simulink model "BlueROVHeavy_SlidingModeControl"  (R2024b)
settings: Solver=ode45  StartTime=0.0  StopTime=T  FixedStep=Ts  RelTol=1e-3
InitFcn:
  | run BlueRovHeavy_init.m;
values from neighbouring files (symbols this model uses):
  BLUEROV_DATA = struct()    [BlueRovHeavy_data.m]
  Ks_D = 25    [BlueRovHeavy_init.m]
  Ks_S = 4    [BlueRovHeavy_init.m]
  Lambda = 21*eye(6)    [BlueRovHeavy_init.m]
libraries: robotcorelib x1
settings Model: Creator=salva  LastModifiedBy=salva

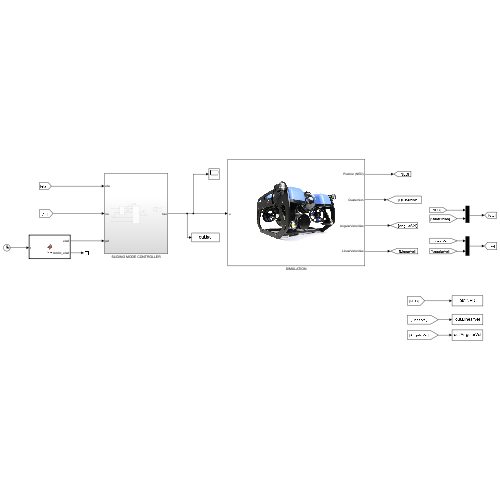
[thumbnail: Simulink's stored preview of the top-level diagram]
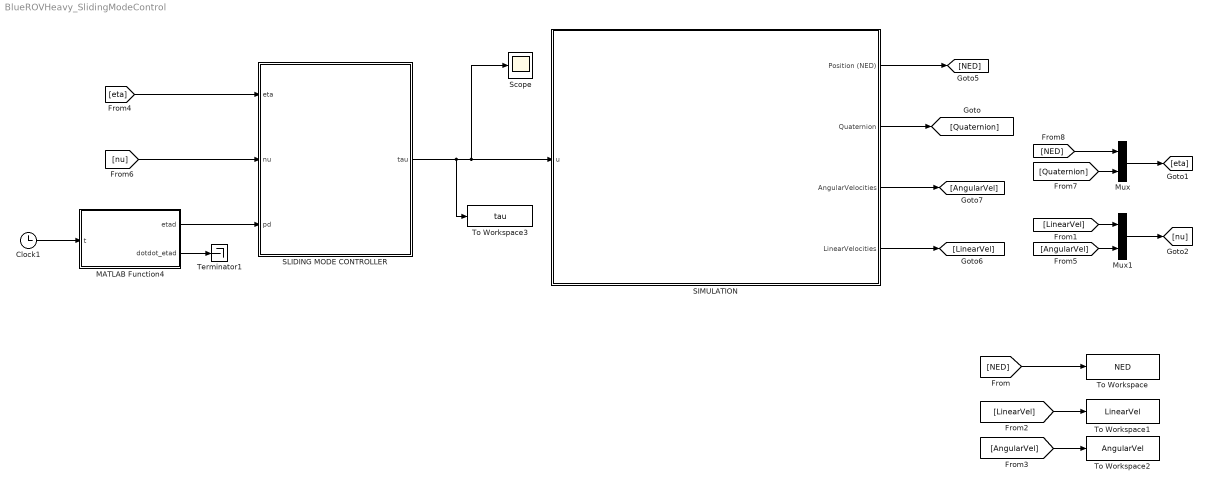
== system BlueROVHeavy_SlidingModeControl ==
  Clock1 : Clock
  MATLAB Function4 : MATLAB Function  TreatAsAtomicUnit=on
  Mux : Mux  Inputs=2
  Mux1 : Mux  Inputs=2
  SIMULATION : Subsystem
      mask Display: image('BlueROVpic.jpg', [0,0,0,0,90,90]);
  SLIDING MODE CONTROLLER : Subsystem
  Scope : Scope
  Terminator1 : Terminator
  To Workspace : ToWorkspace  VariableName=NED  SaveFormat=Timeseries  SampleTime=-1
  To Workspace1 : ToWorkspace  VariableName=LinearVel  SaveFormat=Timeseries  SampleTime=-1
  To Workspace2 : ToWorkspace  VariableName=AngularVel  SaveFormat=Timeseries  SampleTime=-1
  To Workspace3 : ToWorkspace  VariableName=tau  SaveFormat=Timeseries  SampleTime=-1
  wires:
  Mux/1 -> [eta]
  Mux1/1 -> [nu]
  [eta] -> SLIDING MODE CONTROLLER/1(eta)
  [nu] -> SLIDING MODE CONTROLLER/2(nu)
  SLIDING MODE CONTROLLER/1(tau) -> To Workspace3/1, Scope/1, SIMULATION/1(u)
  MATLAB Function4/1(etad) -> SLIDING MODE CONTROLLER/3(pd)
  Clock1/1 -> MATLAB Function4/1(t)
  MATLAB Function4/2(dotdot_etad) -> Terminator1/1
  [NED] -> To Workspace/1
  [AngularVel] -> To Workspace2/1
  [LinearVel] -> To Workspace1/1
  SIMULATION/1(Position (NED)) -> [NED]
  SIMULATION/2(Quaternion) -> [Quaternion]
  [AngularVel] -> Mux1/2
  [LinearVel] -> Mux1/1
  SIMULATION/4(LinearVelocities) -> [LinearVel]
  SIMULATION/3(AngularVelocities) -> [AngularVel]
  [Quaternion] -> Mux/2
  [NED] -> Mux/1

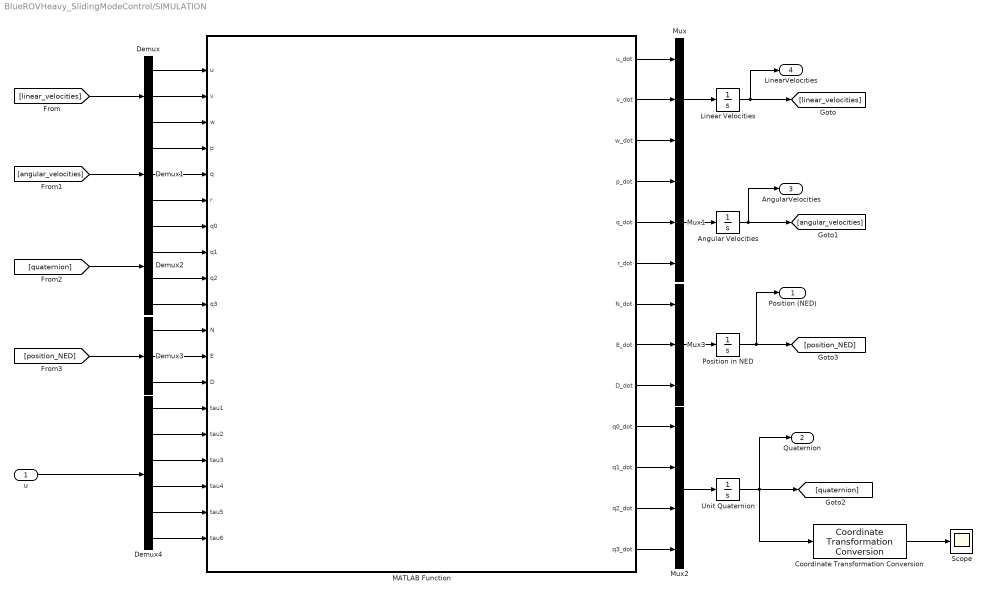
== system BlueROVHeavy_SlidingModeControl/SIMULATION ==
  u : Inport
  Angular Velocities : Integrator  InitialCondition=[0;0;0]  UpperSaturationLimit=50  LowerSaturationLimit=-50
  Coordinate Transformation Conversion : robotcorelib/Coordinate Transformation Conversion  InputRepresentation=Quaternion  InputEulerSequence=ZYX  ShowTrVecInputPort=on  OutputRepresentation=Euler Angles  OutputEulerSequence=XYZ  ShowTrVecOutputPort=on  SimulateUsing=Interpreted execution
  Demux : Demux  Outputs=3
  Demux1 : Demux  Outputs=3
  Demux2 : Demux
  Demux3 : Demux  Outputs=3
  Demux4 : Demux  Outputs=6
  Linear Velocities : Integrator  InitialCondition=[0.1;0;0]
  MATLAB Function : MATLAB Function  TreatAsAtomicUnit=on
  Mux : Mux  Inputs=3
  Mux1 : Mux  Inputs=3
  Mux2 : Mux
  Mux3 : Mux  Inputs=3
  Position in NED : Integrator  InitialCondition=[3;0;9]
  Scope : Scope
  Unit Quaternion : Integrator  InitialCondition=[1,0,0,0]
  Position (NED) : Outport
  Quaternion : Outport  Port=2
  AngularVelocities : Outport  Port=3
  LinearVelocities : Outport  Port=4
  wires:
  Demux1/1 -> MATLAB Function/4(p)
  Demux4/5 -> MATLAB Function/18(tau5)
  Demux1/2 -> MATLAB Function/5(q)
  Demux4/6 -> MATLAB Function/19(tau6)
  Demux/2 -> MATLAB Function/2(v)
  Mux3/1 -> Position in NED/1
  Demux/1 -> MATLAB Function/1(u)
  Demux1/3 -> MATLAB Function/6(r)
  Angular Velocities/1 -> [angular_velocities], AngularVelocities/1
  Demux3/1 -> MATLAB Function/11(N)
  Demux3/3 -> MATLAB Function/13(D)
  Demux4/2 -> MATLAB Function/15(tau2)
  Mux/1 -> Linear Velocities/1
  Mux1/1 -> Angular Velocities/1
  Demux4/4 -> MATLAB Function/17(tau4)
  Demux2/3 -> MATLAB Function/9(q2)
  Demux2/2 -> MATLAB Function/8(q1)
  Demux3/2 -> MATLAB Function/12(E)
  Demux2/1 -> MATLAB Function/7(q0)
  Demux4/1 -> MATLAB Function/14(tau1)
  Demux4/3 -> MATLAB Function/16(tau3)
  Demux/3 -> MATLAB Function/3(w)
  [linear_velocities] -> Demux/1
  [angular_velocities] -> Demux1/1
  [quaternion] -> Demux2/1
  [position_NED] -> Demux3/1
  u/1 -> Demux4/1
  MATLAB Function/1(u_dot) -> Mux/1
  MATLAB Function/2(v_dot) -> Mux/2
  MATLAB Function/3(w_dot) -> Mux/3
  Linear Velocities/1 -> [linear_velocities], LinearVelocities/1
  MATLAB Function/4(p_dot) -> Mux1/1
  MATLAB Function/5(q_dot) -> Mux1/2
  MATLAB Function/6(r_dot) -> Mux1/3
  MATLAB Function/7(N_dot) -> Mux3/1
  MATLAB Function/8(E_dot) -> Mux3/2
  MATLAB Function/9(D_dot) -> Mux3/3
  MATLAB Function/10(q0_dot) -> Mux2/1
  MATLAB Function/11(q1_dot) -> Mux2/2
  MATLAB Function/12(q2_dot) -> Mux2/3
  MATLAB Function/13(q3_dot) -> Mux2/4
  Position in NED/1 -> Position (NED)/1, [position_NED]
  Mux2/1 -> Unit Quaternion/1
  Demux2/4 -> MATLAB Function/10(q3)
  Unit Quaternion/1 -> Quaternion/1, Coordinate Transformation Conversion/1, [quaternion]
  Coordinate Transformation Conversion/1 -> Scope/1

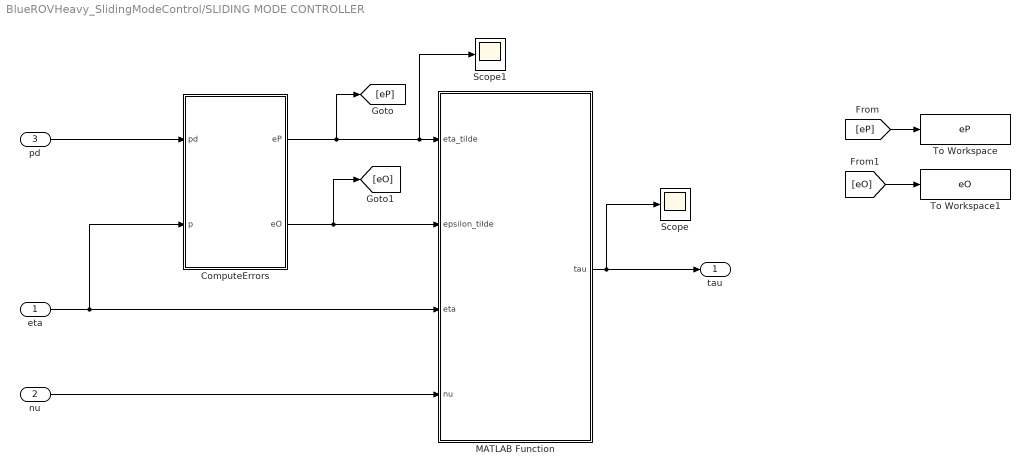
== system BlueROVHeavy_SlidingModeControl/SLIDING MODE CONTROLLER ==
  eta : Inport
  nu : Inport  Port=2
  pd : Inport  Port=3
  ComputeErrors : MATLAB Function  TreatAsAtomicUnit=on
  MATLAB Function : MATLAB Function  TreatAsAtomicUnit=on
  Scope : Scope
  Scope1 : Scope
  To Workspace : ToWorkspace  VariableName=eP  SaveFormat=Timeseries  SampleTime=-1
  To Workspace1 : ToWorkspace  VariableName=eO  SaveFormat=Timeseries  SampleTime=-1
  tau : Outport
  wires:
  pd/1 -> ComputeErrors/1(pd)
  MATLAB Function/1(tau) -> Scope/1, tau/1
  ComputeErrors/2(eO) -> [eO], MATLAB Function/2(epsilon_tilde)
  ComputeErrors/1(eP) -> [eP], Scope1/1, MATLAB Function/1(eta_tilde)
  eta/1 -> ComputeErrors/2(p), MATLAB Function/3(eta)
  nu/1 -> MATLAB Function/4(nu)
  [eO] -> To Workspace1/1
  [eP] -> To Workspace/1

== matlab function BlueROVHeavy_SlidingModeControl/MATLAB Function4 ==
  data: t input; etad output; dotdot_etad output
function [etad,dotdot_etad]  = fcn(t)
% Traiettoria elicoidale 3D con quaternione costante
% etad = [x, y, z, qx, qy, qz, qw]'
% dot_etad = derivata prima
% dotdot_etad = derivata seconda

% Parametri della spirale
r = 4;         % Raggio dell'elica
omega = 0.8;  % Frequenza angolare (rad/s)
vz = 0.6;      % Velocità lungo z

% Posizione elicoidale
x = r * cos(omega * t);
y = r * sin(omega * t);
z = 10+vz * t;

% Derivata prima della posizione
dx = -r * omega * sin(omega * t);
dy =  r * omega * cos(omega * t);
dz = vz;

% Derivata seconda della posizione
ddx = -r * omega^2 * cos(omega * t);
ddy = -r * omega^2 * sin(omega * t);
ddz = 0;

% Quaternione costante (nessuna rotazione)
qx = 1;
qy = 0;
qz = 0;
qw = 0;

% Stato desiderato
etad = [x; y; z; qx; qy; qz; qw];

% Derivata seconda
dotdot_etad = [ddx; ddy; ddz; 0; 0; 0; 0];

end

== matlab function BlueROVHeavy_SlidingModeControl/SIMULATION/MATLAB Function ==
  data: u input; u_dot output; v input; w input; p input; q input; r input; q0 input; q1 input; q2 input; q3 input; N input; E input; D input; tau1 input; tau2 input; tau3 input; tau4 input; tau5 input; tau6 input; v_dot output; w_dot output; p_dot output; q_dot output; r_dot output; N_dot output; E_dot output; D_dot output; q0_dot output; q1_dot output; q2_dot output; q3_dot output; BLUEROV_DATA parameter

function [u_dot, v_dot, w_dot, p_dot, q_dot, r_dot,N_dot,E_dot,D_dot, q0_dot,q1_dot,q2_dot,q3_dot] =  ...
    BlueROV(u, v, w, p, q, r, q0,q1,q2,q3, N, E, D, tau1,tau2,tau3,tau4,tau5,tau6, BLUEROV_DATA)
    
    e1 = BLUEROV_DATA.e1;                    %Body frame unit vector along x
    e2 = BLUEROV_DATA.e2;                    %Body frame unit vector along y
    e3 = BLUEROV_DATA.e3;                    %Body frame unit vector along z
    
    I3 = BLUEROV_DATA.I3;                      %Identity matrix (3x3)
    
    
    m_t = BLUEROV_DATA.m_t;                      %BlueROV mass [Kg]
    W = BLUEROV_DATA.W;                       %Weight [N]
    B = BLUEROV_DATA.B;                       %Boyancy [N]
    r_cb = BLUEROV_DATA.r_cb;                 %Center of boyancy wrt. center of origin [m]
    r_cg = BLUEROV_DATA.r_cg;                %Center of gravity wrt. center of origin [m]
    
    I = BLUEROV_DATA.I;                     %Dyadyic inertia
    SCG =BLUEROV_DATA.SCG;
    
    
    %% Added mass (hydrodynamic derivatives)
    
    X_udot = BLUEROV_DATA.X_udot;   % [kg] 
    Y_vdot = BLUEROV_DATA.Y_vdot;  % [kg]
    Z_wdot = BLUEROV_DATA.Z_wdot; % [kg]
    K_pdot = BLUEROV_DATA.K_pdot;  % [kg m^2/rad]
    M_qdot = BLUEROV_DATA.M_qdot;  % [kg m^2/rad]
    N_rdot = BLUEROV_DATA.N_rdot;  % [kg m^2/rad]
    
    %% Hydrodynamic linear and quadratic damping coefficients
    
    Xu = BLUEROV_DATA.Xu;      % [Ns/m]
    Yv = BLUEROV_DATA.Yv;      % [Ns/m]
    Zw = BLUEROV_DATA.Zw;      % [Ns/m]
    Kp = BLUEROV_DATA.Kp;      % [Ns/rad]
    Mq = BLUEROV_DATA.Mq;      % [Ns/rad]
    Nr = BLUEROV_DATA.Nr;      % [Ns/rad]
    
    Xuu = BLUEROV_DATA.Xuu;    % [Ns^2/m^2]
    Yvv = BLUEROV_DATA.Yvv;    % [Ns^2/m^2]
    Zww = BLUEROV_DATA.Zww;    % [Ns^2/m^2]
    Kpp = BLUEROV_DATA.Kpp;     % [Ns^2/rad^2]
    Mqq = BLUEROV_DATA.Mqq;     % [Ns^2/rad^2]
    Nrr = BLUEROV_DATA.Nrr;     % [Ns^2/rad^2]
    
    
    
    %% Kinematics
    
    Rq=[1-2*(q2^2+q3^2) 2*(q1*q2-q3*q0) 2*(q1*q3+q2*q0);
        2*(q1*q2+q3*q0) 1-2*(q1^2+q3^2) 2*(q2*q3-q1*q0);
        2*(q1*q3-q2*q0) 2*(q2*q3+q1*q0) 1-2*(q1^2+q2^2)];
    Tq=0.5*[-q1,-q2,-q3;
        q0,-q3,q2;
        q3,q0,-q1;
        -q2,q1,q0];

    J_qeta=[Rq,zeros(3,3);zeros(4,3),Tq];
 
    %% Computing Hydrodynamic Damping Matrix D(v)
    epsilon=1e-4;

    D = diag([Xu + Xuu*sqrt(u^2 + epsilon), ...
          Yv + Yvv*sqrt(v^2 + epsilon), ...
          Zw + Zww*sqrt(w^2 + epsilon), ...
          Kp + Kpp*sqrt(p^2 + epsilon), ...
          Mq + Mqq*sqrt(q^2 + epsilon), ...
          Nr + Nrr*sqrt(r^2 + epsilon)]);


    %% Computing Restoring Forces
    
    g_eta = [(-W+B)*(2*q1*q3-2*q2*q0);
            -(W-B)*(2*q2*q3-2*q1*q0);
            (W-B)*(2*q1^2+2*q2^2-1);
            r_cg(3)*W*(2*q2*q3+2*q1*q0);
            r_cg(3)*W*(2*q1*q3-2*q2*q0);
            0];
    
   
    %% Computing Coriolis and Centrifugal Matrix C(v)
     IO = I*[p q r]'; 
     
     S_IO = [0 -IO(3) IO(2);
             IO(3) 0 -IO(1);
            -IO(2) IO(1) 0]; 
             
    S_omega = [0 -r q;
              r 0 -p;
              -q p 0];         
             
       
    C_rb = [m_t*S_omega -m_t*S_omega*SCG;
            m_t*SCG*S_omega -S_IO];
        
    
    C_A = [0 0 0 0 -Z_wdot*w Y_vdot*v;
           0 0 0 -Z_wdot*w 0 -X_udot*u;
           0 0 0 -Y_vdot*v X_udot*u 0;
           0 -Z_wdot*w Y_vdot*v 0 -N_rdot*r M_qdot*q;
           Z_wdot*w 0 -X_udot*u N_rdot*r 0 -K_pdot*p;
           -Y_vdot*v X_udot*u 0 -M_qdot*q K_pdot*p 0];
        
    %% Generalized forces and moments
    tau_c = [tau1 tau2 tau3 tau4 tau5 tau6]';

    %% Total Inertia Matric
    M=BLUEROV_DATA.M;


    %% 6DOF Dynamics and Kinematics
    
    nu_dot=zeros(6,1);
    nu_dot = M\(tau_c-(D+C_rb+C_A)*[u v w p q r]' -g_eta); %6DOF dynamics

    etadot=zeros(7,1); 
    etadot=J_qeta*[u v w p q r]'; %Kinematics
    
    u_dot = nu_dot(1); %Surge velcoity
    v_dot = nu_dot(2); %Sway Velcoity
    w_dot = nu_dot(3); %Heave velocity
    p_dot = nu_dot(4); %Angular velocity around phi
    q_dot = nu_dot(5);  %Angular velcoity around theta
    r_dot = nu_dot(6); %Angular velcoity around psi
  
   
    
    N_dot=etadot(1); % N position
    E_dot=etadot(2); % E position
    D_dot=etadot(3); % D position
    q0_dot=etadot(4); % Quaternion
    q1_dot=etadot(5);
    q2_dot=etadot(6);
    q3_dot=etadot(7);

== matlab function BlueROVHeavy_SlidingModeControl/SLIDING MODE CONTROLLER/ComputeErrors ==
  data: eP output; pd input; eO output; p input
function [eP,eO] = fcn(pd,p)

Qd=pd(4:7);
Qe=p(4:7);

Sd=[0 -Qd(4) Qd(3);
    Qd(4) 0 -Qd(2);
    -Qd(3) Qd(2) 0];

eO=Qe(1)*Qd(2:4)-Qd(1)*Qe(2:4)-Sd*Qe(2:4);

eP=pd(1:3)-p(1:3);

== matlab function BlueROVHeavy_SlidingModeControl/SLIDING MODE CONTROLLER/MATLAB Function ==
  data: eta_tilde input; tau output; epsilon_tilde input; eta input; nu input; BLUEROV_DATA parameter; Ks_S parameter; Ks_D parameter; Lambda parameter
function tau = fcn(eta_tilde,epsilon_tilde,eta,nu, BLUEROV_DATA, Ks_S, Ks_D, Lambda)

     q0=eta(4);q1=eta(5);q2=eta(6);q3=eta(7);

     W = BLUEROV_DATA.W-20;                       %Estimated Weight [N]
     B = BLUEROV_DATA.B-20;                       %Estimated Boyancy [N]
     r_cg = BLUEROV_DATA.r_cg;                %Center of gravity wrt. center of origin [m]
     r_cg(3)=r_cg(3)-0.5;
    
     g_eta = [(-W+B)*(2*q1*q3-2*q2*q0);
                -(W-B)*(2*q2*q3-2*q1*q0);
                (W-B)*(2*q1^2+2*q2^2-1);
                r_cg(3)*W*(2*q2*q3+2*q1*q0);
                r_cg(3)*W*(2*q1*q3-2*q2*q0);
                0];

     Rq=[1-2*(q2^2+q3^2) 2*(q1*q2-q3*q0) 2*(q1*q3+q2*q0);
        2*(q1*q2+q3*q0) 1-2*(q1^2+q3^2) 2*(q2*q3-q1*q0);
        2*(q1*q3-q2*q0) 2*(q2*q3+q1*q0) 1-2*(q1^2+q2^2)];


    
    bandwidth=[0.8;0.8;0.8;1;1;1];
    

    

    s=Lambda*[Rq'*eta_tilde;epsilon_tilde]-nu(:);

    sign_s=zeros(6,1);
    for i=1:6
        if s(i)>bandwidth(i)
            sign_s(i)=1;
        elseif s(i)<-bandwidth(i)
            sign_s(i)=-1;
        else
            sign_s(i)=s(i)/bandwidth(i);
        end

    end
    
    % tau=KD*s+g_eta+KS*sign(s-bandwidth);
    tau=Ks_D*s+g_eta+Ks_S*sign_s;
